simulink model "modelBraccioSimulation"  (R2021a)
settings: Solver=VariableStepAuto  StartTime=0.0  StopTime=inf  RelTol=1e-3
values from neighbouring files (symbols this model uses):
  adMotorLimits = [ 0, 180 ... (first row only)    [initSim.m]
  adWaypoints = ppval(aTrajectory, adX)    [initSim.m]
  adWeight = [0 0 0 1 1 1]    [initSim.m]    (also in validatorScript.m)
undefined symbols (not defined in the file or in its folder): Levenberg, Marquardt
libraries: vrlib x3, robotcorelib x2, robotmaniplib x2
settings Model: Creator=angelo  LastModifiedBy=angelo

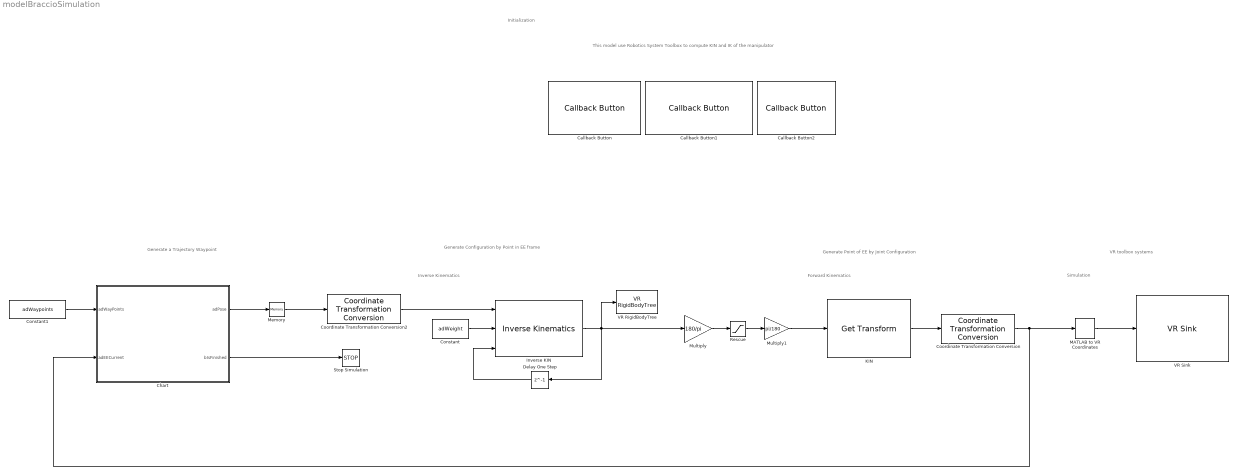
== system modelBraccioSimulation ==
  note: Generate a Trajectory Waypoint
  note: Initialization
  note: Generate Point of EE by Joint Configuration
  note: Forward Kinematics
  note: Inverse Kinematics
  note: Simulation
  note: This model use Robotics System Toolbox to compute KIN and IK of the manipulator
  note: Generate Configuration by Point in EE frame
  note: VR toolbox systems
  Callback Button : CallbackButton  ButtonText=Load Robot Model
      settings: ClickFcn=|
      | % Take a rigidBodyTree Object from URDF file
      | oRbtBraccio = importrobot('Tinkerkit_model/tinkerkit.urdf');
      | 
      | oRbtBraccio.Bodies{1}.Joint.HomePosition = pi/2;
      | oRbtBraccio.Bodies{2}.Joint.HomePosition = pi/2;
      | oRbtBraccio.Bodies{3}.Joint.HomePosition = pi/2;
      | oRbtBraccio.Bodies{4}.Joint.HomePosition = pi/2;
      | oRbtBraccio.Bodies{5}.Joint.HomePosition = 0;
      | oRbtBraccio.Bodies{8}.Joint.HomePosition = 73 * pi / 180;
      | 
      | % Add EE
      | adEEOffset = 0.16;
      | oRbtEE     = robotics.RigidBody('ee');
      | setFixedTransform(oRbtEE.Joint, trvec2tform([0 0 adEEOffset]));
      | addBody(oRbtBraccio, oRbtEE, 'link4');
  Callback Button1 : CallbackButton  ButtonText=Load Motor Limits and Weights
      settings: ClickFcn=|
      | % Weight for IK block
      | adWeight     = [0 0 0 1 1 1];
      | 
      | % Motor Limits
      | adMotorLimits = [ 0, 180;
      |                  15, 165;
      |                   0, 180;
      |                   0, 180;
      |                   0, 180;
      |                  10,  73;
      | ];
  Callback Button2 : CallbackButton  ButtonText=Load WayPoints
      settings: ClickFcn=|
      | % Waypoints
      | adStartPoint = [0 0 0.4515];
      | adBallPoint  = [0.1 0.2 0.05];
      | adPoint      = [0.15 0 0.25];
      | adGoalPoint  = [0.1 -0.2 0.05];
      | 
      | adWaypoints  = [adStartPoint;
      |                 adBallPoint;
      |                 adPoint;
      |                 adGoalPoint;];
      | 
      | % Generate Trajectory from points
      | aTrajectory = cscvn(adWaypoints');
      | nNumPoints = size(adWaypoints, 1);
      | adX = linspace(0, aTrajectory.breaks(end), nNumPoints * 20);
      | 
      | % Total points for EE
      | adWaypoints = ppval(aTrajectory, adX);
  Chart : Stateflow chart  TreatAsAtomicUnit=on
  Constant : Constant  Value=adWeight
  Constant1 : Constant  Value=adWaypoints
  Coordinate Transformation Conversion : robotcorelib/Coordinate Transformation Conversion  InputRepresentation=Homogeneous Transformation  InputEulerSequence=ZYX  ShowTrVecInputPort=on  OutputRepresentation=Translation Vector  OutputEulerSequence=ZYX  ShowTrVecOutputPort=on  SimulateUsing=Interpreted execution
      settings: SourceProductBaseCode=NV,RO,RR,UV
  Coordinate Transformation Conversion2 : robotcorelib/Coordinate Transformation Conversion  InputRepresentation=Translation Vector  InputEulerSequence=ZYX  ShowTrVecInputPort=on  OutputRepresentation=Homogeneous Transformation  OutputEulerSequence=ZYX  ShowTrVecOutputPort=on  SimulateUsing=Interpreted execution
      settings: SourceProductBaseCode=NV,RO,RR,UV
  Delay One Step : Delay  DelayLength=1  InitialCondition=zeros(6, 1)
  Inverse KIN : robotmaniplib/Inverse Kinematics  RigidBodyTree=oRbtBraccio  EndEffector=ee  ShowInfo=off  SolverName=Levenberg-Marquardt  EnforceJointLimits=on  MaxIterations=1500  MaxTime=10  GradientTolerance=1e-7  SolutionTolerance=1e-6  StepTolerance=1e-14  ErrorChangeTolerance=1e-12  UseErrorDamping=on  DampingBias=0.0025  SimulateUsing=Interpreted execution
  KIN : robotmaniplib/Get Transform  RigidBodyTree=oRbtBraccio  SourceBody=ee  TargetBody=base_link  SimulateUsing=Interpreted execution
  MATLAB to VR Coordinates : vrlib/Utilities/MATLAB to VR Coordinates
      settings: SourceProductBaseCode=SL
  Memory : Memory
  Multiply : Gain  Gain=180/pi
  Multiply1 : Gain  Gain=pi/180
  Rescue : Saturate  UpperLimit=adMotorLimits(:,2)  LowerLimit=adMotorLimits(:,1)
  Stop Simulation : Stop
  VR RigidBodyTree : vrlib/VR RigidBodyTree  VrmlFile=/home/angelo/1.PROJECTS/arm-manipulator-6dof/graphics/robotWorld.x3d  RBT=oRbtBraccio  useRBT=off  Ts=-1  ForceViewerOpen=off
      settings: SourceProductBaseCode=SL
  VR Sink : vrlib/VR Sink  InstantiateOnLoad=on  SampleTime=0.1  ViewEnable=on  RemoteChange=off  RemoteView=off  FieldsWritten=SetPoint.translation.3.1.1.double  WorldFileName=graphics/robotWorld.x3d  AutoView=on  VideoDimensions=[]  AllowVariableSize=off
  wires:
  Delay One Step/1 -> Inverse KIN/3
  Inverse KIN/1 -> VR RigidBodyTree/1, Multiply/1, Delay One Step/1
  KIN/1 -> Coordinate Transformation Conversion/1
  MATLAB to VR Coordinates/1 -> VR Sink/1
  Coordinate Transformation Conversion/1 -> MATLAB to VR Coordinates/1, Chart/2(adEECurrent)
  Constant/1 -> Inverse KIN/2
  Multiply/1 -> Rescue/1
  Rescue/1 -> Multiply1/1
  Multiply1/1 -> KIN/1
  Coordinate Transformation Conversion2/1 -> Inverse KIN/1
  Chart/2(bIsFinished) -> Stop Simulation/1
  Chart/1(adPose) -> Memory/1
  Memory/1 -> Coordinate Transformation Conversion2/1
  Constant1/1 -> Chart/1(adWayPoints)

== stateflow chart modelBraccioSimulation/Chart ==
  settings: executeAtInitialization=1
  (default) -> (junction 3) : {adError = vecnorm((adPose - adEECurrent), 2, 1);}
  (junction 3) -> (junction 7) [order 1] : [all(adError < tol)]
  (junction 7) -> (junction 11) [order 1] : [i == length(adWayPoints)]
  (junction 3) -> (junction 22) [order 2]
  (junction 7) -> (junction 17) [order 2] : {i = i + 1;}
  (junction 11) -> (junction 14) : {bIsFinished = true;}
  (junction 17) -> (junction 22)
  (junction 14) -> (junction 17)
  (junction 22) -> (junction 26) : { adPose = adWayPoints(:, i) ; }
  data: adWayPoints input; adEECurrent input; adError local; tol local =.01; adPose output =adStartPoint'; bIsFinished output =false; i local =1
